simulink model "manual"  (R2020b)
settings: Solver=VariableStepAuto  StartTime=0.0  StopTime=10.0  RelTol=1e-3
settings Model: Creator=Jose  LastModifiedBy=Jose

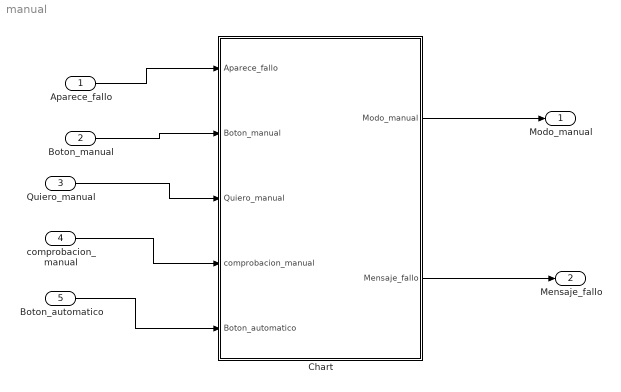
== system manual ==
  Aparece_fallo : Inport  OutDataTypeStr=boolean  PortDimensions=1
  Boton_manual : Inport  Port=2  OutDataTypeStr=boolean  PortDimensions=1
  Quiero_manual : Inport  Port=3  OutDataTypeStr=boolean  PortDimensions=1
  comprobacion_manual : Inport  Port=4  OutDataTypeStr=boolean  PortDimensions=1
  Boton_automatico : Inport  Port=5  OutDataTypeStr=boolean  PortDimensions=1
  Chart : Stateflow chart  TreatAsAtomicUnit=on
  Modo_manual : Outport  OutDataTypeStr=boolean  PortDimensions=1
  Mensaje_fallo : Outport  Port=2  OutDataTypeStr=boolean  PortDimensions=1
  wires:
  Aparece_fallo/1 -> Chart/1(Aparece_fallo)
  Boton_manual/1 -> Chart/2(Boton_manual)
  Quiero_manual/1 -> Chart/3(Quiero_manual)
  comprobacion_manual/1 -> Chart/4(comprobacion_manual)
  Boton_automatico/1 -> Chart/5(Boton_automatico)
  Chart/1(Modo_manual) -> Modo_manual/1
  Chart/2(Mensaje_fallo) -> Mensaje_fallo/1

== stateflow chart manual/Chart ==
  state Control_Automatico
    en:
    Mensaje_fallo=false;
    Modo_manual=false;
  state Manual_fallo
    en:
    Mensaje_fallo=true;
    Modo_manual=false;
  state Pregunta_seguridad
    en:
    Mensaje_fallo=false;
    Modo_manual=false
  state Control_Manual
    en:
    Modo_manual=true;
  (default) -> Control_Automatico
  Control_Manual -> Control_Automatico [order 2] : [Boton_automatico & ~Aparece_fallo]
  Control_Automatico -> Control_Automatico [order 1] : [(~Aparece_fallo & ~Boton_manual)]
  Control_Automatico -> Manual_fallo [order 2] : [Aparece_fallo]
  Control_Automatico -> Pregunta_seguridad [order 3] : [Boton_manual]
  Pregunta_seguridad -> Pregunta_seguridad [order 1] : [~comprobacion_manual]
  Manual_fallo -> Manual_fallo [order 1] : [~Quiero_manual]
  Manual_fallo -> Control_Manual [order 2] : [Quiero_manual]
  Pregunta_seguridad -> Control_Manual [order 2] : [comprobacion_manual]
  Control_Manual -> Control_Manual [order 1] : [~Boton_automatico || Aparece_fallo]
  data: Aparece_fallo input; Boton_manual input; Quiero_manual input; comprobacion_manual input; Boton_automatico input; Modo_manual output; Mensaje_fallo output
